simulink model "modi1_6"  (R2022b)
settings: Solver=VariableStepAuto  StartTime=0.0  StopTime=100.0  RelTol=1e-3
values from neighbouring files (symbols this model uses):
  a0 = 0.00447127    [modi1.m]
  a1 = 0.108205    [modi1.m]
  a2 = 0.683702    [modi1.m]
  alfa1 = 1.2    [modi1.m]
  alfa2 = 0.56    [modi1.m]
  alfa3 = -1.45    [modi1.m]
  alfa4 = 1.15    [modi1.m]
  b0 = 0.00201207    [modi1.m]
  u_lin = 0.5    [modi1.m]
settings Model: Creator=zalew  LastModifiedBy=zalew

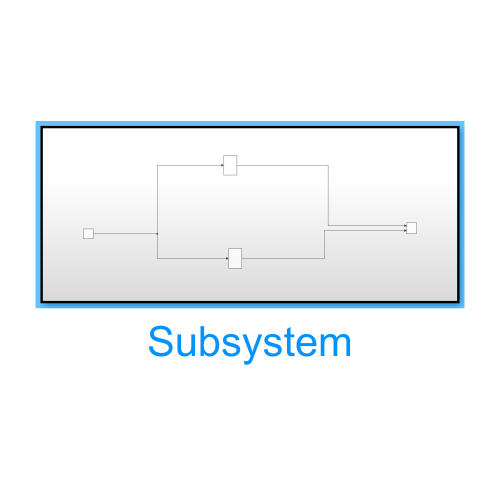
[thumbnail: Simulink's stored preview of the top-level diagram]
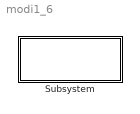
== system modi1_6 ==
  Subsystem : Subsystem

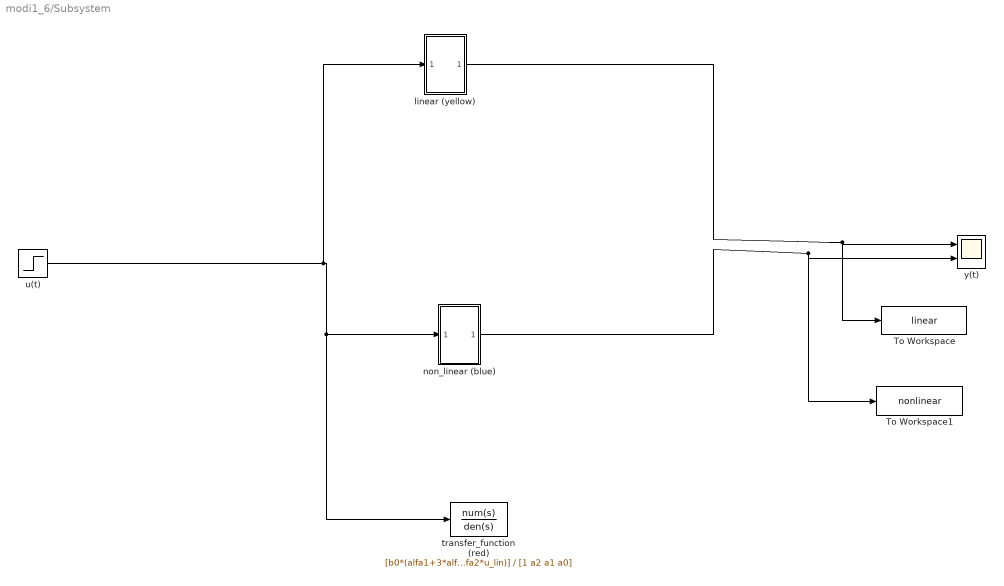
== system modi1_6/Subsystem ==
  To Workspace : ToWorkspace  VariableName=linear  SaveFormat=Structure With Time  SampleTime=-1
  To Workspace1 : ToWorkspace  VariableName=nonlinear  SaveFormat=Structure With Time  SampleTime=-1
  linear (yellow) : Subsystem
  non_linear (blue) : Subsystem
  transfer_function (red) : TransferFcn  Numerator=[b0*(alfa1+3*alfa3*u_lin^2+4*alfa4*u_lin^3+2*alfa2*u_lin)]  Denominator=[1 a2 a1 a0]
  u(t) : Step  Time=10  After=0.9  SampleTime=0
  y(t) : Scope  NumInputPorts=2
  wires:
  u(t)/1 -> linear (yellow)/1(u(t)1), transfer_function (red)/1, non_linear (blue)/1(u(t)2)
  non_linear (blue)/1(y(t)2) -> To Workspace1/1, y(t)/2
  linear (yellow)/1(y(t)1) -> To Workspace/1, y(t)/1

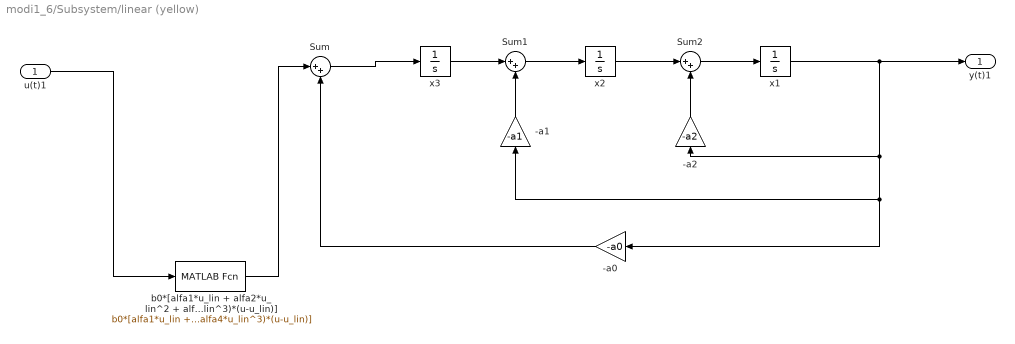
== system modi1_6/Subsystem/linear (yellow) ==
  u(t)1 : Inport
  -a0 : Gain  Gain=-a0
  -a1 : Gain  Gain=-a1
  -a2 : Gain  Gain=-a2
  Sum : Sum  Inputs=|++
  Sum1 : Sum  Inputs=|++
  Sum2 : Sum  Inputs=|++
  b0*[alfa1*u_lin + alfa2*u_lin^2 + alfa3*u_lin^3 + alfa4*u_lin^4 + (alfa1 + 2*alfa2*u_lin + 3*alfa3*u_lin^2 + 4*alfa4*u_lin^3)*(u-u_lin)] : MATLABFcn  MATLABFcn=b0*[alfa1*u_lin + alfa2*u_lin^2 + alfa3*u_lin^3 + alfa4*u_lin^4 + (alfa1 + 2*alfa2*u_lin + 3*alfa3*u_lin^2 + 4*alfa4*u_lin^3)*(u-u_lin)]
  x1 : Integrator
  x2 : Integrator
  x3 : Integrator
  y(t)1 : Outport
  wires:
  b0*[alfa1*u_lin + alfa2*u_lin^2 + alfa3*u_lin^3 + alfa4*u_lin^4 + (alfa1 + 2*alfa2*u_lin + 3*alfa3*u_lin^2 + 4*alfa4*u_lin^3)*(u-u_lin)]/1 -> Sum/1
  x1/1 -> y(t)1/1, -a2/1, -a1/1, -a0/1
  x3/1 -> Sum1/1
  -a2/1 -> Sum2/2
  -a1/1 -> Sum1/2
  Sum2/1 -> x1/1
  u(t)1/1 -> b0*[alfa1*u_lin + alfa2*u_lin^2 + alfa3*u_lin^3 + alfa4*u_lin^4 + (alfa1 + 2*alfa2*u_lin + 3*alfa3*u_lin^2 + 4*alfa4*u_lin^3)*(u-u_lin)]/1
  Sum1/1 -> x2/1
  -a0/1 -> Sum/2
  Sum/1 -> x3/1
  x2/1 -> Sum2/1

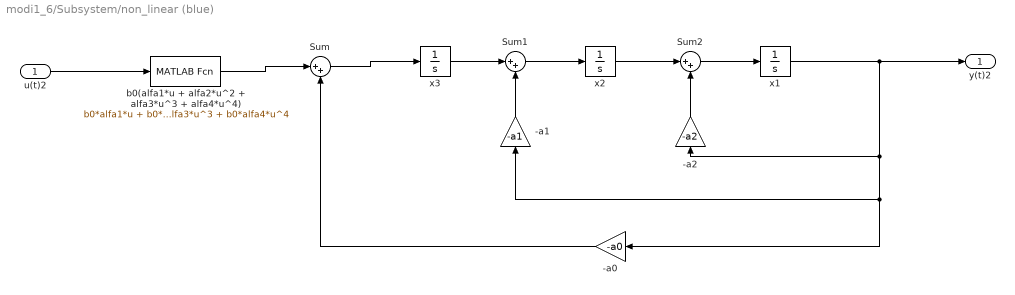
== system modi1_6/Subsystem/non_linear (blue) ==
  u(t)2 : Inport
  -a0 : Gain  Gain=-a0
  -a1 : Gain  Gain=-a1
  -a2 : Gain  Gain=-a2
  Sum : Sum  Inputs=|++
  Sum1 : Sum  Inputs=|++
  Sum2 : Sum  Inputs=|++
  b0(alfa1*u + alfa2*u^2 + alfa3*u^3 + alfa4*u^4) : MATLABFcn  MATLABFcn=b0*alfa1*u + b0*alfa2*u^2 + b0*alfa3*u^3 + b0*alfa4*u^4
  x1 : Integrator
  x2 : Integrator
  x3 : Integrator
  y(t)2 : Outport
  wires:
  -a1/1 -> Sum1/2
  b0(alfa1*u + alfa2*u^2 + alfa3*u^3 + alfa4*u^4)/1 -> Sum/1
  Sum1/1 -> x2/1
  x1/1 -> y(t)2/1, -a2/1, -a1/1, -a0/1
  -a0/1 -> Sum/2
  Sum/1 -> x3/1
  u(t)2/1 -> b0(alfa1*u + alfa2*u^2 + alfa3*u^3 + alfa4*u^4)/1
  -a2/1 -> Sum2/2
  Sum2/1 -> x1/1
  x3/1 -> Sum1/1
  x2/1 -> Sum2/1
